simulink model "OpenLoopAngular"  (R2019a)
settings: Solver=VariableStepAuto  StartTime=0.0  StopTime=10.0  RelTol=1e-3
values from neighbouring files (symbols this model uses):
  den1 = [taum 1]    [classical.m]
  Kdin = (2*zetacin*wcin*Tm-1)/Km    [classical.m]
  Kpin = wcin^2*Tm/(Kdin*Km)    [classical.m]
  num1 = [Km1]    [classical.m]
settings Model: Creator=xde12  LastModifiedBy=xde12

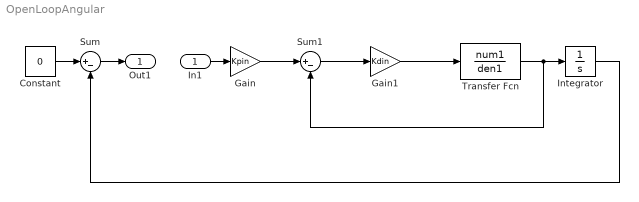
== system OpenLoopAngular ==
  In1 : Inport
  Constant : Constant  Value=0
  Gain : Gain  Gain=Kpin
  Gain1 : Gain  Gain=Kdin
  Integrator : Integrator
  Sum : Sum  Inputs=|+-
  Sum1 : Sum  Inputs=|+-
  Transfer Fcn : TransferFcn  Numerator=num1  Denominator=den1
  Out1 : Outport
  wires:
  Constant/1 -> Sum/1
  Gain/1 -> Sum1/1
  Sum1/1 -> Gain1/1
  Gain1/1 -> Transfer Fcn/1
  Transfer Fcn/1 -> Sum1/2, Integrator/1
  Integrator/1 -> Sum/2
  Sum/1 -> Out1/1
  In1/1 -> Gain/1
